simulink model "sampleModel1958"  (R2023a)
settings: Solver=VariableStepAuto  StartTime=0.0  StopTime=10.0  RelTol=1e-3
libraries: hdlsllib x8, simulink x3
settings Model: Creator=user1  LastModifiedBy=user1

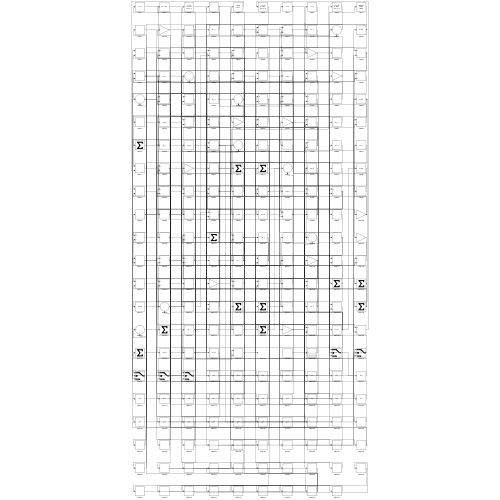
[thumbnail: Simulink's stored preview of the top-level diagram]
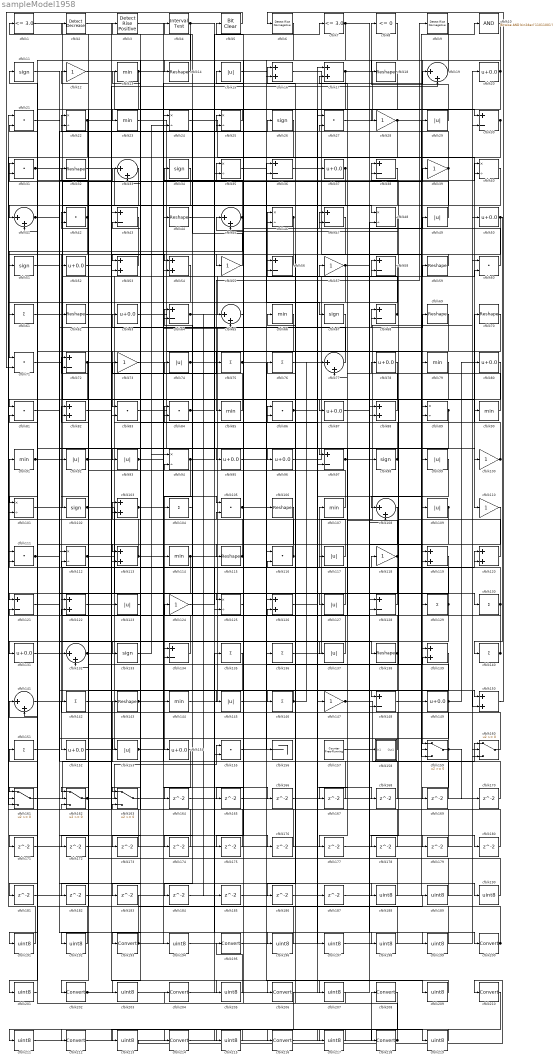
== system sampleModel1958 ==
  cfblk1 : hdlsllib/Logic and Bit Operations/Compare To Constant  relop=<=  const=3.0  OutDataTypeStr=boolean
  cfblk10 : simulink/Logic and Bit Operations/Bitwise Operator  logicop=AND  UseBitMask=on  BitMask=bin2dec('11011001')  BitMaskRealWorld=Stored Integer
      settings: LibrarySourceBlock=|
      | hdlsllib/Logic and Bit
      | Operations/Bitwise
      | Operator
  cfblk{12,28,39,55,57,73,100,110,118,124,147} (11 alike) : Gain
  cfblk{22,24..25,35,40,46,48,89,94,101,112,125} (12 alike) : Product  Inputs=*/  RndMeth=Zero  SaturateOnIntegerOverflow=on
  cfblk{11,26,34,51,67,98,102,133} (8 alike) : Signum
  cfblk{16..17,53..54,82,88,103,113,119..120,122,126,139,150} (14 alike) : Sum
  cfblk{61,75..76,104,129..130,135..136,140,142,146,151} (12 alike) : Sum  Inputs=+
  cfblk{21,27,31,42,60,71,81,83..84,86,105,111,116,155} (14 alike) : DotProduct  OutDataTypeStr=Inherit: Inherit via internal rule
  cfblk{14,18,32,44,59,62,69..70,106,115,138,143} (12 alike) : Reshape
  cfblk{13,23,66,79,85,90..91,107,114,144} (10 alike) : MinMax
  cfblk{19,33,41,45,65,77,108,132,141} (9 alike) : Sum  Inputs=|++
  cfblk{15,29,49,74,92..93,99,109,117,123,127,137,145,153} (14 alike) : Abs  SaturateOnIntegerOverflow=off
  cfblk{30,36,38,43,47,56,58,64,68,72,97,121,128,134,148} (15 alike) : Sum  Inputs=+-
  cfblk{20,37,50,52,63,78,80,87,95..96,131,149,152,154} (14 alike) : Bias  Bias=0.0  SaturateOnIntegerOverflow=off
  cfblk156 : Terminator
  cfblk157 : hdlsllib/Sources/Counter Free-Running  NumBits=16  tsamp=-1
  cfblk158 : Subsystem
      settings: LibrarySourceBlock=|
      | hdlsllib/Ports &
      | Subsystems/Subsystem
  cfblk{159..163} (5 alike) : Switch  SaturateOnIntegerOverflow=off  InputSameDT=off
  cfblk{164..187} (24 alike) : Delay  SampleTime=1
  cfblk{188..192,194,196..199,201,203,205,207,209,211,213,215,217,219} (20 alike) : DataTypeConversion  OutDataTypeStr=uint8  SaturateOnIntegerOverflow=off  RndMeth=Floor
  cfblk{193,195,200,202,204,206,208,210,212,214,216,218} (12 alike) : DataTypeConversion  SaturateOnIntegerOverflow=off  RndMeth=Floor
  cfblk2 : simulink/Logic and Bit Operations/Detect Decrease  vinit=0.0  OutDataTypeStr=boolean
      settings: LibrarySourceBlock=|
      | hdlsllib/Logic and Bit
      | Operations/Detect
      | Decrease
  cfblk3 : hdlsllib/Logic and Bit Operations/Detect Rise Positive  vinit=0  OutDataTypeStr=boolean
  cfblk4 : hdlsllib/Logic and Bit Operations/Interval Test  IntervalClosedRight=on  uplimit=0.5  IntervalClosedLeft=on  lowlimit=-0.5  OutDataTypeStr=boolean
  cfblk5 : simulink/Logic and Bit Operations/Bit Clear  iBit=0
      settings: LibrarySourceBlock=|
      | hdlsllib/Logic and Bit
      | Operations/Bit Clear
  cfblk6 : hdlsllib/Logic and Bit Operations/Detect Rise Nonnegative  vinit=0  OutDataTypeStr=boolean
  cfblk7 : hdlsllib/Logic and Bit Operations/Compare To Constant  relop=<=  const=3.0  OutDataTypeStr=boolean
  cfblk8 : hdlsllib/Logic and Bit Operations/Compare To Zero  relop=<=  OutDataTypeStr=boolean
  cfblk9 : hdlsllib/Logic and Bit Operations/Detect Rise Nonnegative  vinit=0  OutDataTypeStr=boolean
  wires:
  cfblk40/1 -> cfblk159/1
  cfblk133/1 -> cfblk94/1
  cfblk144/1 -> cfblk68/1
  cfblk147/1 -> cfblk160/1, cfblk108/2
  cfblk152/1 -> cfblk57/1
  cfblk56/1 -> cfblk55/1
  cfblk53/1 -> cfblk152/1
  cfblk45/1 -> cfblk71/1, cfblk34/1
  cfblk74/1 -> cfblk9/1, cfblk89/2
  cfblk158/1(Out1) -> cfblk5/1
  cfblk129/1 -> cfblk45/1, cfblk141/2
  cfblk10/1 -> cfblk149/1
  cfblk112/1 -> cfblk130/1, cfblk38/1
  cfblk94/1 -> cfblk154/1, cfblk7/1
  cfblk59/1 -> cfblk53/1
  cfblk19/1 -> cfblk14/1
  cfblk66/1 -> cfblk83/1
  cfblk50/1 -> cfblk140/1, cfblk186/1
  cfblk98/1 -> cfblk86/1, cfblk64/1
  cfblk128/1 -> cfblk91/1
  cfblk69/1 -> cfblk85/1
  cfblk37/1 -> cfblk41/1, cfblk161/3
  cfblk65/1 -> cfblk125/1
  cfblk146/1 -> cfblk144/1, cfblk77/1
  cfblk5/1 -> cfblk71/2
  cfblk63/1 -> cfblk79/1
  cfblk148/1 -> cfblk10/1
  cfblk16/1 -> cfblk99/1
  cfblk54/1 -> cfblk81/1
  cfblk60/1 -> cfblk35/1
  cfblk24/1 -> cfblk110/1
  cfblk1/1 -> cfblk83/2
  cfblk38/1 -> cfblk134/1
  cfblk114/1 -> cfblk37/1, cfblk153/1
  cfblk100/1 -> cfblk70/1, cfblk33/2
  cfblk127/1 -> cfblk12/1
  cfblk68/1 -> cfblk46/1, cfblk27/2
  cfblk91/1 -> cfblk96/1, cfblk129/1, cfblk26/1
  cfblk18/1 -> cfblk104/1
  cfblk101/1 -> cfblk39/1
  cfblk150/1 -> cfblk6/1
  cfblk77/1 -> cfblk63/1
  cfblk131/1 -> cfblk107/1
  cfblk23/1 -> cfblk95/1
  cfblk95/1 -> cfblk40/1
  cfblk43/1 -> cfblk52/1
  cfblk159/1 -> cfblk76/1, cfblk169/1, cfblk170/1
  cfblk138/1 -> cfblk145/1, cfblk94/2, cfblk72/2
  cfblk96/1 -> cfblk59/1
  cfblk107/1 -> cfblk42/1
  cfblk115/1 -> cfblk3/1, cfblk72/1
  cfblk161/1 -> cfblk143/1
  cfblk46/1 -> cfblk122/1, cfblk172/1
  cfblk39/1 -> cfblk115/1, cfblk22/1
  cfblk17/1 -> cfblk30/1, cfblk41/2
  cfblk4/1 -> cfblk133/1, cfblk198/1
  cfblk136/1 -> cfblk60/1
  cfblk34/1 -> cfblk61/1
  cfblk86/1 -> cfblk16/1, cfblk109/1
  cfblk109/1 -> cfblk183/1, cfblk184/1
  cfblk36/1 -> cfblk90/1
  cfblk25/1 -> cfblk23/1
  cfblk162/1 -> cfblk155/1, cfblk19/2, cfblk118/1
  cfblk82/1 -> cfblk123/1
  cfblk124/1 -> cfblk117/1
  cfblk139/1 -> cfblk146/1
  cfblk62/1 -> cfblk43/1
  cfblk13/1 -> cfblk92/1, cfblk28/1
  cfblk160/1 -> cfblk82/1
  cfblk6/1 -> cfblk16/2
  cfblk12/1 -> cfblk158/1(In1)
  cfblk117/1 -> cfblk73/1
  cfblk141/1 -> cfblk98/1
  cfblk15/1 -> cfblk48/1
  cfblk92/1 -> cfblk36/1, cfblk75/1
  cfblk51/1 -> cfblk97/1
  cfblk140/1 -> cfblk78/1, cfblk77/2
  cfblk104/1 -> cfblk84/1
  cfblk29/1 -> cfblk8/1
  cfblk32/1 -> cfblk46/2
  cfblk11/1 -> cfblk132/1
  cfblk120/1 -> cfblk45/2
  cfblk113/1 -> cfblk103/1, cfblk65/2
  cfblk70/1 -> cfblk155/2
  cfblk90/1 -> cfblk31/1
  cfblk20/1 -> cfblk97/2, cfblk18/1
  cfblk28/1 -> cfblk159/2, cfblk121/1
  cfblk83/1 -> cfblk156/1
  cfblk99/1 -> cfblk108/1
  cfblk26/1 -> cfblk53/2
  cfblk163/1 -> cfblk116/1
  cfblk78/1 -> cfblk162/1
  cfblk151/1 -> cfblk200/1
  cfblk75/1 -> cfblk86/2, cfblk100/1
  cfblk49/1 -> cfblk31/2
  cfblk145/1 -> cfblk56/1
  cfblk137/1 -> cfblk112/2
  cfblk64/1 -> cfblk58/1, cfblk150/2, cfblk185/1
  cfblk52/1 -> cfblk137/1
  cfblk8/1 -> cfblk134/2
  cfblk116/1 -> cfblk74/1, cfblk25/2
  cfblk89/1 -> cfblk131/1, cfblk127/1, cfblk148/2
  cfblk157/1 -> cfblk49/1
  cfblk132/1 -> cfblk69/1, cfblk124/1
  cfblk149/1 -> cfblk162/2, cfblk103/2, cfblk65/1, cfblk38/2, cfblk80/1, cfblk101/2
  cfblk73/1 -> cfblk105/1
  cfblk134/1 -> cfblk122/2
  cfblk119/1 -> cfblk163/1
  cfblk57/1 -> cfblk111/2, cfblk64/2, cfblk199/1
  cfblk85/1 -> cfblk13/1
  cfblk79/1 -> cfblk93/1
  cfblk143/1 -> cfblk84/2, cfblk19/1
  cfblk27/1 -> cfblk29/1
  cfblk31/1 -> cfblk114/1, cfblk54/2
  cfblk35/1 -> cfblk67/1
  cfblk55/1 -> cfblk4/1
  cfblk71/1 -> cfblk159/3
  cfblk102/1 -> cfblk147/1, cfblk192/1
  cfblk72/1 -> cfblk60/2, cfblk181/1
  cfblk61/1 -> cfblk35/2
  cfblk130/1 -> cfblk58/2, cfblk121/2
  cfblk118/1 -> cfblk47/1, cfblk175/1, cfblk177/1, cfblk201/1
  cfblk88/1 -> cfblk17/2
  cfblk41/1 -> cfblk62/1, cfblk33/1, cfblk101/1
  cfblk14/1 -> cfblk1/1
  cfblk30/1 -> cfblk128/2, cfblk113/2
  cfblk93/1 -> cfblk40/2, cfblk173/1
  cfblk22/1 -> cfblk54/1, cfblk161/2
  cfblk135/1 -> cfblk202/1
  cfblk106/1 -> cfblk193/1
  cfblk7/1 -> cfblk119/1, cfblk191/1
  cfblk48/1 -> cfblk102/1
  cfblk84/1 -> cfblk125/2, cfblk87/1
  cfblk97/1 -> cfblk47/2, cfblk179/1
  cfblk103/1 -> cfblk24/2, cfblk166/1
  cfblk153/1 -> cfblk44/1, cfblk120/2
  cfblk58/1 -> cfblk113/1
  cfblk42/1 -> cfblk11/1, cfblk51/1
  cfblk125/1 -> cfblk25/1
  cfblk121/1 -> cfblk148/1
  cfblk105/1 -> cfblk136/1, cfblk150/1
  cfblk155/1 -> cfblk139/2
  cfblk111/1 -> cfblk138/1, cfblk68/2
  cfblk108/1 -> cfblk161/1
  cfblk122/1 -> cfblk120/1
  cfblk154/1 -> cfblk164/1
  cfblk164/1 -> cfblk160/2
  cfblk9/1 -> cfblk165/1
  cfblk165/1 -> cfblk119/2
  cfblk166/1 -> cfblk56/2
  cfblk110/1 -> cfblk167/1
  cfblk167/1 -> cfblk24/1
  cfblk76/1 -> cfblk168/1
  cfblk168/1 -> cfblk112/1
  cfblk169/1 -> cfblk82/2
  cfblk170/1 -> cfblk116/2
  cfblk67/1 -> cfblk171/1
  cfblk171/1 -> cfblk139/1
  cfblk172/1 -> cfblk42/2
  cfblk173/1 -> cfblk162/3
  cfblk47/1 -> cfblk174/1
  cfblk174/1 -> cfblk132/2
  cfblk175/1 -> cfblk163/3
  cfblk81/1 -> cfblk176/1
  cfblk176/1 -> cfblk111/1
  cfblk177/1 -> cfblk160/3
  cfblk80/1 -> cfblk178/1
  cfblk178/1 -> cfblk43/2
  cfblk179/1 -> cfblk163/2
  cfblk87/1 -> cfblk180/1
  cfblk180/1 -> cfblk128/1
  cfblk181/1 -> cfblk17/1
  cfblk33/1 -> cfblk182/1
  cfblk182/1 -> cfblk36/2
  cfblk184/1 -> cfblk30/2
  cfblk185/1 -> cfblk89/1
  cfblk186/1 -> cfblk88/2
  cfblk187/1 -> cfblk48/2
  cfblk2/1 -> cfblk188/1
  cfblk188/1 -> cfblk15/1
  cfblk183/1 -> cfblk189/1
  cfblk189/1 -> cfblk2/1
  cfblk21/1 -> cfblk190/1
  cfblk190/1 -> cfblk27/1
  cfblk191/1 -> cfblk21/1
  cfblk192/1 -> cfblk21/2
  cfblk193/1 -> cfblk22/2, cfblk20/1
  cfblk3/1 -> cfblk194/1
  cfblk194/1 -> cfblk106/1
  cfblk44/1 -> cfblk196/1
  cfblk196/1 -> cfblk142/1
  cfblk126/1 -> cfblk197/1
  cfblk197/1 -> cfblk50/1
  cfblk198/1 -> cfblk126/1
  cfblk199/1 -> cfblk126/2
  cfblk200/1 -> cfblk32/1, cfblk81/2
  cfblk201/1 -> cfblk151/1
  cfblk202/1 -> cfblk187/1, cfblk88/1
  cfblk123/1 -> cfblk203/1
  cfblk203/1 -> cfblk135/1
  cfblk142/1 -> cfblk205/1
  cfblk205/1 -> cfblk195/1
  cfblk195/1 -> cfblk207/1
  cfblk207/1 -> cfblk204/1
  cfblk204/1 -> cfblk209/1
  cfblk209/1 -> cfblk206/1
  cfblk206/1 -> cfblk211/1
  cfblk211/1 -> cfblk208/1
  cfblk208/1 -> cfblk213/1
  cfblk213/1 -> cfblk210/1
  cfblk210/1 -> cfblk215/1
  cfblk215/1 -> cfblk212/1
  cfblk216/1 -> cfblk218/1
  cfblk212/1 -> cfblk217/1
  cfblk217/1 -> cfblk214/1
  cfblk218/1 -> cfblk141/1, cfblk105/2, cfblk66/1
  cfblk214/1 -> cfblk219/1
  cfblk219/1 -> cfblk216/1

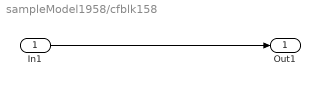
== system sampleModel1958/cfblk158 ==
  In1 : Inport
  Out1 : Outport
  wires:
  In1/1 -> Out1/1
